simulink model "practica1ejercicio8"  (Simulink 7.5)
settings: Solver=ode45  StartTime=0.0  StopTime=10.0  RelTol=1e-3
settings Model: Creator=Mariano  LastModifiedBy=Mariano

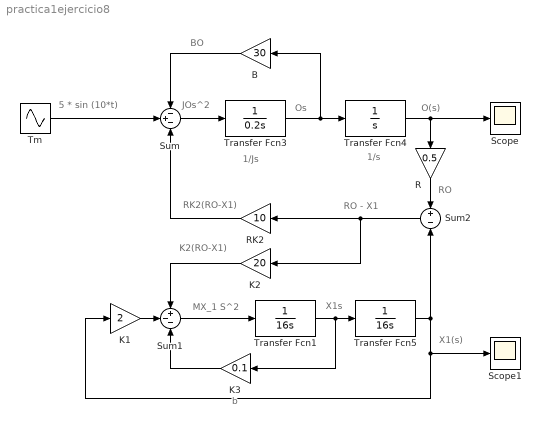
== system practica1ejercicio8 ==
  note: 5 * sin (10*t)
  note: JOs^2
  note: BO
  note: RK2(RO-X1)
  note: O(s)
  note: RO
  note: X1(s)
  note: 1/Js
  note: Os
  note: 1/s
  note: RO - X1
  note: K2(RO-X1)
  note: MX_1 S^2
  note: X1s
  note: b
  B : Gain  Gain=30  ParameterDataType=fixdt(1, 16)  ParameterScaling=2^0  OutDataType=fixdt(1, 16)  OutScaling=2^0
  K1 : Gain  Gain=2  ParameterDataType=fixdt(1, 16)  ParameterScaling=2^0  OutDataType=fixdt(1, 16)  OutScaling=2^0
  K2 : Gain  Gain=20  ParameterDataType=fixdt(1, 16)  ParameterScaling=2^0  OutDataType=fixdt(1, 16)  OutScaling=2^0
  K3 : Gain  Gain=0.1  ParameterDataType=fixdt(1, 16)  ParameterScaling=2^0  OutDataType=fixdt(1, 16)  OutScaling=2^0
  R : Gain  Gain=0.5  ParameterDataType=fixdt(1, 16)  ParameterScaling=2^0  OutDataType=fixdt(1, 16)  OutScaling=2^0
  RK2 : Gain  Gain=10  ParameterDataType=fixdt(1, 16)  ParameterScaling=2^0  OutDataType=fixdt(1, 16)  OutScaling=2^0
  Scope : Scope
  Scope1 : Scope
  Sum : Sum  Inputs=-+-  OutDataType=fixdt(1, 16)  OutScaling=2^0
  Sum1 : Sum  Inputs=+--  OutDataType=fixdt(1, 16)  OutScaling=2^0
  Sum2 : Sum  Inputs=+|-  OutDataType=fixdt(1, 16)  OutScaling=2^0
  Tm : Sin  Amplitude=5  Bias=0  Frequency=10  Phase=0  Samples=10  SampleTime=0  Offset=0
  Transfer Fcn1 : TransferFcn  Denominator=[16 0]
  Transfer Fcn3 : TransferFcn  Denominator=[0.2 0]
  Transfer Fcn4 : TransferFcn  Denominator=[1 0]
  Transfer Fcn5 : TransferFcn  Denominator=[16 0]
  wires:
  Tm/1 -> Sum/2
  K2/1 -> Sum1/1
  K1/1 -> Sum1/2
  Transfer Fcn5/1 -> Sum2/2, Scope1/1, K1/1
  B/1 -> Sum/1
  RK2/1 -> Sum/3
  R/1 -> Sum2/1
  Sum2/1 -> RK2/1, K2/1
  Sum/1 -> Transfer Fcn3/1
  Transfer Fcn4/1 -> R/1, Scope/1
  Transfer Fcn3/1 -> Transfer Fcn4/1, B/1
  Sum1/1 -> Transfer Fcn1/1
  Transfer Fcn1/1 -> Transfer Fcn5/1, K3/1
  K3/1 -> Sum1/3
